simulink model "CONTROL_LQR_DISCRETO"  (R2017b)
settings: Solver=VariableStepAuto  StartTime=0.0  StopTime=10.0  RelTol=1e-3
values from neighbouring files (symbols this model uses):
  K = dlqr(F,G,Q,R)    [ESPACIODEESTADOS.m]    (also in lqr_digital.m = dlqr(Ad,Bd,Q,R))
undefined symbols (not defined in the file or in its folder): Ad, Bd, Cd, Dd, DiscIntNeverNeededParam
libraries: simulink x2
settings Model: Creator=Gustavo  LastModifiedBy=Gustavo

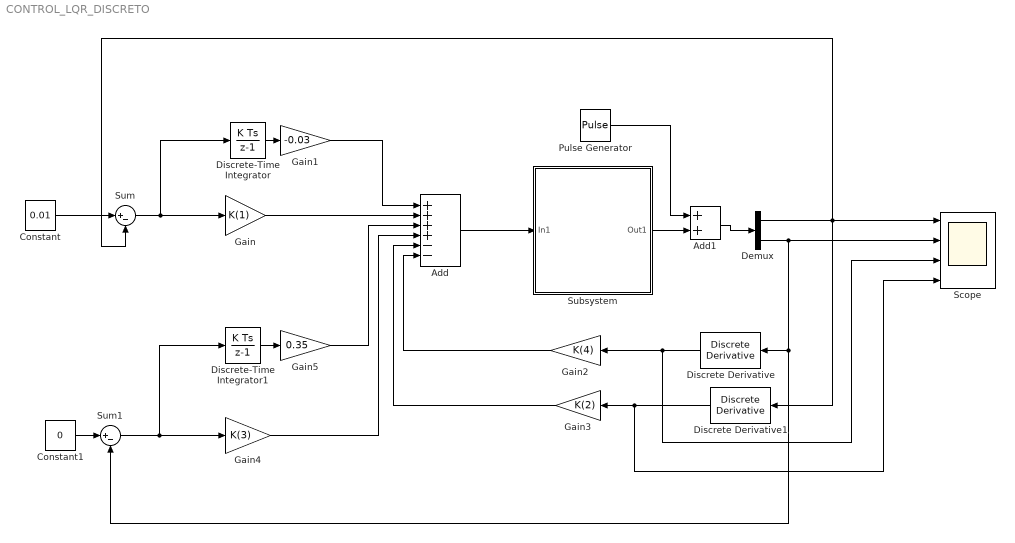
== system CONTROL_LQR_DISCRETO ==
  Add : Sum  Inputs=++++--
  Add1 : Sum
  Constant : Constant  Value=0.01
  Constant1 : Constant  Value=0
  Demux : Demux  Outputs=2
  Discrete Derivative : simulink/Discrete/Discrete Derivative  gainval=1.0  ICPrevScaledInput=0.0  OutMin=[]  OutMax=[]  OutDataType=fixdt(1, 16)  OutScaling=2^-10  DoSatur=off
  Discrete Derivative1 : simulink/Discrete/Discrete Derivative  gainval=1.0  ICPrevScaledInput=0.0  OutMin=[]  OutMax=[]  OutDataType=fixdt(1, 16)  OutScaling=2^-10  DoSatur=off
  Discrete-Time Integrator : DiscreteIntegrator  InitialConditionSetting=State (most efficient)  SampleTime=0.005  ICPrevOutput=DiscIntNeverNeededParam  ICPrevScaledInput=DiscIntNeverNeededParam
  Discrete-Time Integrator1 : DiscreteIntegrator  InitialConditionSetting=State (most efficient)  SampleTime=0.005  ICPrevOutput=DiscIntNeverNeededParam  ICPrevScaledInput=DiscIntNeverNeededParam
  Gain : Gain  Gain=K(1)
  Gain1 : Gain  Gain=-0.03
  Gain2 : Gain  Gain=K(4)
  Gain3 : Gain  Gain=K(2)
  Gain4 : Gain  Gain=K(3)
  Gain5 : Gain  Gain=0.35
  Pulse Generator : DiscretePulseGenerator  PulseType=Time based  Amplitude=0.01  Period=1  PhaseDelay=1
  Scope : Scope  NumInputPorts=4
  Subsystem : Subsystem
      mask Display: image('C:\Users\Gustavo\Desktop\invertedpendulum.jpg');
  Sum : Sum  Inputs=|+-
  Sum1 : Sum  Inputs=|+-
  wires:
  Constant/1 -> Sum/1
  Constant1/1 -> Sum1/1
  Demux/1 -> Discrete Derivative1/1, Scope/1, Sum/2
  Demux/2 -> Sum1/2, Discrete Derivative/1, Scope/2
  Sum/1 -> Discrete-Time Integrator/1, Gain/1
  Discrete Derivative/1 -> Scope/3, Gain2/1
  Discrete Derivative1/1 -> Gain3/1, Scope/4
  Gain3/1 -> Add/5
  Gain2/1 -> Add/6
  Discrete-Time Integrator/1 -> Gain1/1
  Gain1/1 -> Add/1
  Gain4/1 -> Add/4
  Gain/1 -> Add/2
  Discrete-Time Integrator1/1 -> Gain5/1
  Sum1/1 -> Gain4/1, Discrete-Time Integrator1/1
  Gain5/1 -> Add/3
  Add/1 -> Subsystem/1(In1)
  Add1/1 -> Demux/1
  Subsystem/1(Out1) -> Add1/2
  Pulse Generator/1 -> Add1/1

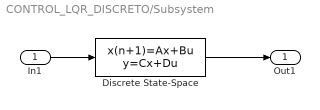
== system CONTROL_LQR_DISCRETO/Subsystem ==
  In1 : Inport
  Discrete State-Space : DiscreteStateSpace  A=Ad  B=Bd  C=Cd  D=Dd  SampleTime=0.005
  Out1 : Outport
  wires:
  In1/1 -> Discrete State-Space/1
  Discrete State-Space/1 -> Out1/1
